simulink model "simulink19"  (R2018a)
settings: Solver=ode4  StartTime=0.0  StopTime=15.0  FixedStep=1e-4  RelTol=1e-3
libraries: simulink x1
settings Model: Creator=User  LastModifiedBy=User

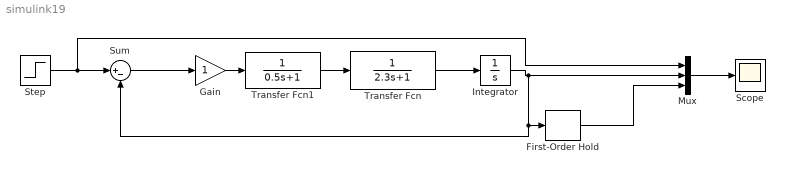
== system simulink19 ==
  First-Order Hold : simulink/Discrete/First-Order Hold  DisableCoverage=on  Ts=1
      settings: SourceProductName=Simulink  SourceProductBaseCode=SL
  Gain : Gain
  Integrator : Integrator
  Mux : Mux  Inputs=3
  Scope : Scope
  Step : Step  Time=0  SampleTime=0
  Sum : Sum  Inputs=|+-
  Transfer Fcn : TransferFcn  Denominator=[2.3 1]
  Transfer Fcn1 : TransferFcn  Denominator=[0.5 1]
  wires:
  Transfer Fcn/1 -> Integrator/1
  Sum/1 -> Gain/1
  Step/1 -> Mux/1, Sum/1
  Gain/1 -> Transfer Fcn1/1
  Integrator/1 -> First-Order Hold/1, Sum/2, Mux/2
  Mux/1 -> Scope/1
  Transfer Fcn1/1 -> Transfer Fcn/1
  First-Order Hold/1 -> Mux/3
